simulink model "Task_Es"  (R2022b)
settings: Solver=ode45  StartTime=0.0  StopTime=10.0  RelTol=1e-3
undefined symbols (not defined in the file): A, absolute_encoder_counts_per_revolution, B, C, C_pid, Cz_zoh, init, Jgain, K_ctr_sine, K_I_sine, theta_l_init, vision_fps, w
libraries: simulink_extras x16
settings Model: Creator=tumisangramotlhwa  LastModifiedBy=tumisangramotlhwa

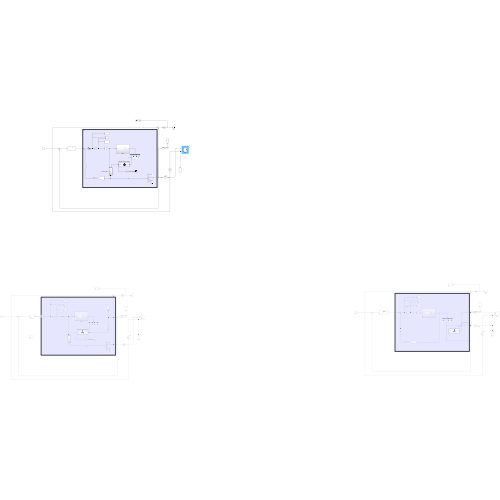
[thumbnail: Simulink's stored preview of the top-level diagram]
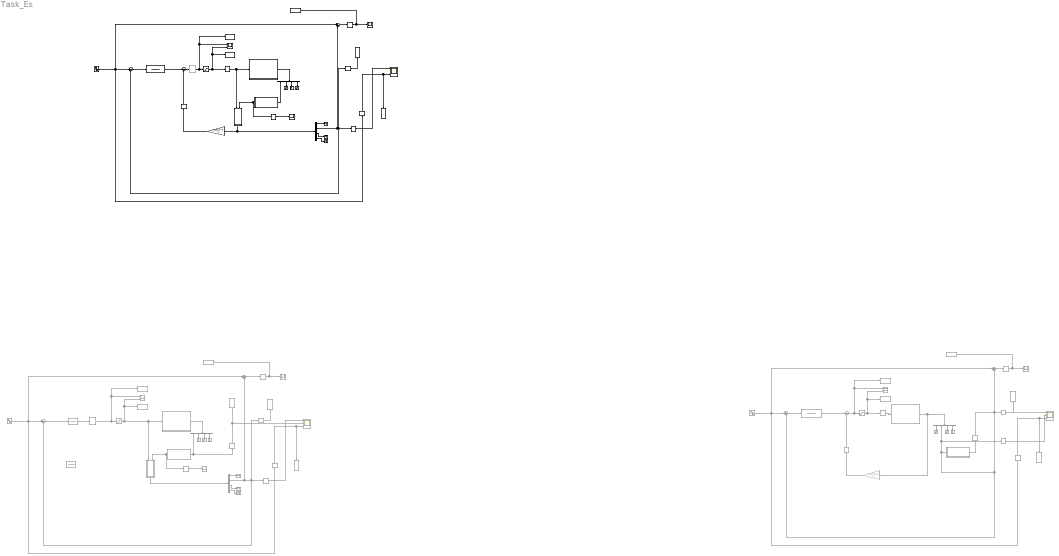
== system Task_Es ==
  note: G(s)
  note: G(s)
  note: G(s)
  AbsoluteEncoderSensorInterface1 : Subsystem  TreatAsAtomicUnit=on
      mask Display: image('$imagefile'); % Use "Edit Image" on toolstrip to change.
  AbsoluteEncoderSensorInterface2 : Subsystem  Commented=on  TreatAsAtomicUnit=on
      mask Display: image('$imagefile'); % Use "Edit Image" on toolstrip to change.
  C(s) : TransferFcn  Commented=on  Numerator=C_pid.Numerator{1,1}  Denominator=C_pid.Denominator{1,1}
  C(z) ZOH : DiscreteTransferFcn  Commented=on  Numerator=Cz_zoh.Numerator{1,1}  Denominator=Cz_zoh.Denominator{1,1}
  Demux1 : Demux
  Demux2 : Demux
  Demux3 : Demux  Commented=on
  Demux4 : Demux  Commented=on
  Demux5 : Demux  Commented=on
  K1 : Gain  Gain=K_ctr_sine  Multiplication=Matrix(K*u) (u vector)
  K2 : Gain  Commented=on  Gain=K_ctr_sine  Multiplication=Matrix(K*u) (u vector)
  Luenberger Observer : Subsystem  TreatAsAtomicUnit=on
  Luenberger Observer1 : Subsystem  Commented=on  TreatAsAtomicUnit=on
  Memory1 : Memory  Commented=on
  Memory2 : Memory
  Memory3 : Memory
  Memory4 : Memory  Commented=on
  PLANT1 : Subsystem
  PLANT2 : Subsystem  Commented=on
  PLANT3 : Subsystem  Commented=on
  Radians to Degrees{7..17} (11 alike) : simulink_extras/Transformations/Radians to Degrees  Commented=on
  Radians to Degrees{2..6} (5 alike) : simulink_extras/Transformations/Radians to Degrees
  Rate Transition : RateTransition  Commented=through  OutPortSampleTime=1/50
  Rate Transition1 : RateTransition  Commented=on  OutPortSampleTime=1/50
  Saturation1 : Saturate  UpperLimit=6  LowerLimit=-6
  Saturation2 : Saturate  Commented=on  UpperLimit=6  LowerLimit=-6
  Saturation3 : Saturate  Commented=on  UpperLimit=6  LowerLimit=-6
  Scope : Scope
  Scope1 : Scope  NumInputPorts=2
  Scope2 : Scope  Commented=on
  Scope3 : Scope  Commented=on  NumInputPorts=2
  Scope4 : Scope  Commented=on  NumInputPorts=2
  Sine Wave1 : Sin  Amplitude=deg2rad(20)  Frequency=pi/2  Phase=deg2rad(20)  SampleTime=0
  Sine Wave2 : Sin  Commented=on  Amplitude=deg2rad(20)  Frequency=pi/2  Phase=deg2rad(20)  SampleTime=0
  Sine Wave3 : Sin  Commented=on  Amplitude=deg2rad(20)  Frequency=pi/2  Phase=deg2rad(20)  SampleTime=0
  Sum{1,5,7..8} (4 alike) : Sum  Commented=on  Inputs=|+-
  Sum2 : Sum  Inputs=|+-
  Sum3 : Sum  Commented=on  Inputs=|--
  Sum4 : Sum  Inputs=|--
  Sum6 : Sum  Inputs=|+-
  Terminator{1..2,9..15} (9 alike) : Terminator  Commented=on
  Terminator{3..8} (6 alike) : Terminator
  To File1 : ToFile  Filename=Error.mat  MatrixName=Error  SaveFormat=Timeseries
  To File10 : ToFile  Commented=on  Filename=trueu.mat  MatrixName=trueu  SaveFormat=Timeseries
  To File11 : ToFile  Commented=on  Filename=truth.mat  MatrixName=truth  SaveFormat=Timeseries
  To File12 : ToFile  Commented=on  Filename=Error.mat  MatrixName=Error  SaveFormat=Timeseries
  To File13 : ToFile  Commented=on  Filename=reference.mat  MatrixName=reference  SaveFormat=Timeseries
  To File14 : ToFile  Commented=on  Filename=y.mat  MatrixName=y  SaveFormat=Timeseries
  To File15 : ToFile  Commented=on  Filename=commandu.mat  MatrixName=commandu  SaveFormat=Timeseries
  To File16 : ToFile  Commented=on  Filename=trueu.mat  MatrixName=trueu  SaveFormat=Timeseries
  To File2 : ToFile  Commented=on  Filename=Error.mat  MatrixName=Error  SaveFormat=Timeseries
  To File3 : ToFile  Commented=on  Filename=reference.mat  MatrixName=reference  SaveFormat=Timeseries
  To File4 : ToFile  Commented=on  Filename=y.mat  MatrixName=y  SaveFormat=Timeseries
  To File5 : ToFile  Commented=on  Filename=commandu.mat  MatrixName=commandu  SaveFormat=Timeseries
  To File6 : ToFile  Filename=reference.mat  MatrixName=reference  SaveFormat=Timeseries
  To File7 : ToFile  Filename=y.mat  MatrixName=y  SaveFormat=Timeseries
  To File8 : ToFile  Filename=commandu.mat  MatrixName=commandu  SaveFormat=Timeseries
  To File9 : ToFile  Filename=trueu.mat  MatrixName=trueu  SaveFormat=Timeseries
  Transfer Fcn : TransferFcn  Numerator=[K_I_sine]  Denominator=[1 0 w^2]
  Transfer Fcn1 : TransferFcn  Commented=on  Numerator=[K_I_sine]  Denominator=[1 0 w^2]
  VisionSensorInterface : Subsystem  Commented=on  TreatAsAtomicUnit=on
      mask Display: image('$imagefile'); % Use "Edit Image" on toolstrip to change.
  error1 : Scope  Commented=on
  error2 : Scope
  error3 : Scope  Commented=on
  scope1 : Scope  NumInputPorts=3
  scope2 : Scope  Commented=on  NumInputPorts=3
  scope3 : Scope  Commented=on  NumInputPorts=3
  wires:
  Luenberger Observer/1(x_hat) -> Demux2/1, K1/1  "x_hat"
  K1/1 -> Memory2/1  "K*x_hat"
  Memory3/1 -> Luenberger Observer/1(u), PLANT1/1(u)
  Demux2/4 -> Terminator7/1
  Transfer Fcn/1 -> Sum4/1
  PLANT1/1(x) -> Demux1/1
  Demux2/3 -> Terminator8/1
  Demux1/2 -> Terminator4/1
  Sum2/1 -> Transfer Fcn/1  "error"
  Memory2/1 -> Sum4/2
  Demux1/4 -> Terminator6/1
  Radians to Degrees5/1 -> scope1/3, To File6/1  "reference"
  Radians to Degrees4/1 -> To File7/1  "sensor measurement"
  Demux1/3 -> Terminator5/1
  Saturation1/1 -> Memory3/1, To File9/1, Scope1/2  "true input"
  Demux2/2 -> Radians to Degrees6/1, Radians to Degrees4/1, Sum2/2, Sum6/2  "link angle"
  Demux2/1 -> Terminator3/1
  Sum4/1 -> Rate Transition/1  "command input"
  Sine Wave1/1 -> Sum6/1, Radians to Degrees5/1, Sum2/1  "y"
  Radians to Degrees2/1 -> Scope/1  "sensor measurement"
  Radians to Degrees3/1 -> To File1/1, error2/1
  Sum6/1 -> Radians to Degrees3/1
  Radians to Degrees6/1 -> scope1/1  "link angle"
  K2/1 -> Memory1/1  "K*x_hat"
  PLANT2/1(x) -> Demux3/1, K2/1
  Demux3/3 -> Terminator9/1
  Demux3/4 -> Terminator10/1
  Sum5/1 -> Radians to Degrees9/1
  Radians to Degrees7/1 -> scope2/1  "sensor measurement"
  Radians to Degrees9/1 -> To File2/1, error1/1
  Transfer Fcn1/1 -> Sum3/1
  Saturation2/1 -> Memory4/1, To File10/1, Scope3/2  "true input"
  Sum3/1 -> Saturation2/1, To File5/1, Scope3/1  "command input"
  Sum1/1 -> Transfer Fcn1/1  "error"
  Radians to Degrees10/1 -> To File4/1  "sensor measurement"
  Memory1/1 -> Sum3/2
  Sine Wave2/1 -> Sum5/1, Radians to Degrees11/1, Sum1/1  "y"
  Demux3/2 -> Radians to Degrees8/1, Sum5/2, Radians to Degrees10/1, Sum1/2, VisionSensorInterface/1(y_plant)  "link angle"
  Memory4/1 -> PLANT2/1(u)
  Radians to Degrees11/1 -> scope2/3, To File3/1  "reference"
  Demux3/1 -> Terminator2/1
  VisionSensorInterface/1(y_vision) -> Radians to Degrees7/1
  Radians to Degrees8/1 -> scope2/2  "link angle"
  Rate Transition/1 -> Saturation1/1, To File8/1, Scope1/1
  AbsoluteEncoderSensorInterface1/1(y_absenc) -> Luenberger Observer/2(y), Radians to Degrees2/1
  Demux1/1 -> AbsoluteEncoderSensorInterface1/1(y_plant)
  Demux5/3 -> Terminator15/1
  Luenberger Observer1/1(x_hat) -> Demux5/1  "x_hat"
  AbsoluteEncoderSensorInterface2/1(y_absenc) -> Luenberger Observer1/2(y), Radians to Degrees13/1
  Radians to Degrees17/1 -> scope3/1  "link angle"
  Saturation3/1 -> Luenberger Observer1/1(u), PLANT3/1(u), To File16/1, Scope4/2  "true input"
  Radians to Degrees14/1 -> To File12/1, error3/1
  Demux5/2 -> Radians to Degrees17/1, Radians to Degrees15/1, Sum7/2, Sum8/2  "link angle"
  Radians to Degrees13/1 -> Scope2/1  "sensor measurement"
  Demux4/1 -> Radians to Degrees12/1, AbsoluteEncoderSensorInterface2/1(y_plant)
  PLANT3/1(x) -> Demux4/1
  Rate Transition1/1 -> Saturation3/1, To File15/1, Scope4/1
  Sum8/1 -> Radians to Degrees14/1
  Sine Wave3/1 -> Sum8/1, Radians to Degrees16/1, Sum7/1  "y"
  Demux5/4 -> Terminator14/1
  Demux4/2 -> Terminator11/1
  Demux4/4 -> Terminator13/1
  Demux4/3 -> Terminator12/1
  Radians to Degrees16/1 -> scope3/3, To File13/1  "reference"
  Radians to Degrees12/1 -> To File11/1, scope3/2  "ground truth"
  Demux5/1 -> Terminator1/1
  Radians to Degrees15/1 -> To File14/1  "sensor measurement"
  C(s)/1 -> Rate Transition1/1  "command input"
  Sum7/1 -> C(s)/1  "error"

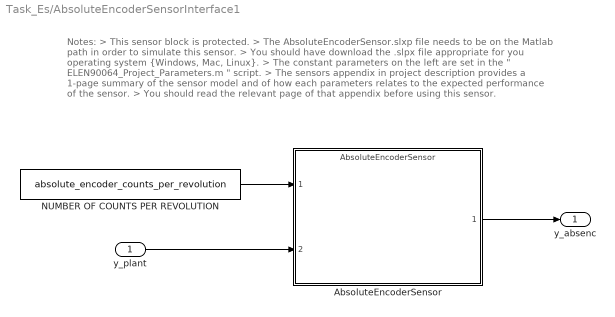
== system Task_Es/AbsoluteEncoderSensorInterface1 ==
  note: Notes:
      | > This sensor block is protected.
      | > The AbsoluteEncoderSensor.slxp file needs to be on the Matlab path in order to simulate this sensor.
      | > You should have download the .slpx file appropriate for you operating system {Windows, Mac, Linux}.
      | > The constant parameters on the left are set in the " ELEN90064_Project_Parameters.m " script.
      | > The sensors appendix in project description provides a 1-page summary of the sensor model and of how each parameters relates to the expected performance of the sensor.
      | > You should read the relevant page of that appendix before using this sensor.
  y_plant : Inport
  AbsoluteEncoderSensor : ModelReference  ModelNameDialog=AbsoluteEncoderSensor.slxp  ModelReferenceVersion=1.16  CopyOfModelProtected=on
  NUMBER OF COUNTS PER REVOLUTION : Constant  Value=absolute_encoder_counts_per_revolution
  y_absenc : Outport
  wires:
  NUMBER OF COUNTS PER REVOLUTION/1 -> AbsoluteEncoderSensor/1
  y_plant/1 -> AbsoluteEncoderSensor/2
  AbsoluteEncoderSensor/1 -> y_absenc/1

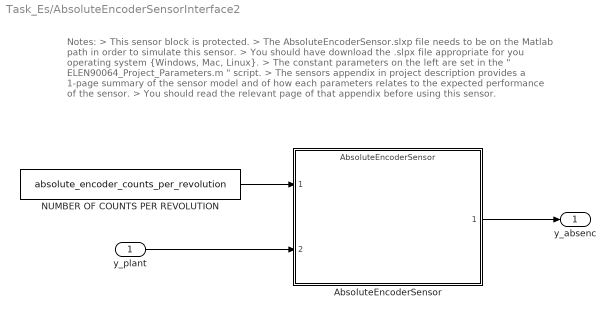
== system Task_Es/AbsoluteEncoderSensorInterface2 ==
  note: Notes:
      | > This sensor block is protected.
      | > The AbsoluteEncoderSensor.slxp file needs to be on the Matlab path in order to simulate this sensor.
      | > You should have download the .slpx file appropriate for you operating system {Windows, Mac, Linux}.
      | > The constant parameters on the left are set in the " ELEN90064_Project_Parameters.m " script.
      | > The sensors appendix in project description provides a 1-page summary of the sensor model and of how each parameters relates to the expected performance of the sensor.
      | > You should read the relevant page of that appendix before using this sensor.
  y_plant : Inport
  AbsoluteEncoderSensor : ModelReference  ModelNameDialog=AbsoluteEncoderSensor.slxp  ModelReferenceVersion=1.16  CopyOfModelProtected=on
  NUMBER OF COUNTS PER REVOLUTION : Constant  Value=absolute_encoder_counts_per_revolution
  y_absenc : Outport
  wires:
  NUMBER OF COUNTS PER REVOLUTION/1 -> AbsoluteEncoderSensor/1
  y_plant/1 -> AbsoluteEncoderSensor/2
  AbsoluteEncoderSensor/1 -> y_absenc/1

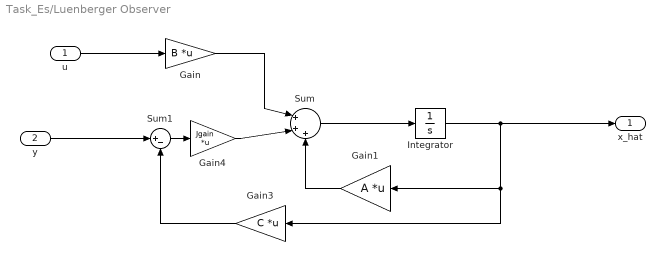
== system Task_Es/Luenberger Observer ==
  u : Inport
  y : Inport  Port=2
  Gain : Gain  Gain=B  Multiplication=Matrix(K*u) (u vector)
  Gain1 : Gain  Gain=A  Multiplication=Matrix(K*u) (u vector)
  Gain3 : Gain  Gain=C  Multiplication=Matrix(K*u) (u vector)
  Gain4 : Gain  Gain=Jgain  Multiplication=Matrix(K*u) (u vector)
  Integrator : Integrator
  Sum : Sum  Inputs=|+++
  Sum1 : Sum  Inputs=|+-
  x_hat : Outport
  wires:
  Gain/1 -> Sum/1
  Gain4/1 -> Sum/2
  Sum1/1 -> Gain4/1
  Gain3/1 -> Sum1/2
  Gain1/1 -> Sum/3
  Sum/1 -> Integrator/1
  Integrator/1 -> x_hat/1, Gain1/1, Gain3/1
  u/1 -> Gain/1
  y/1 -> Sum1/1

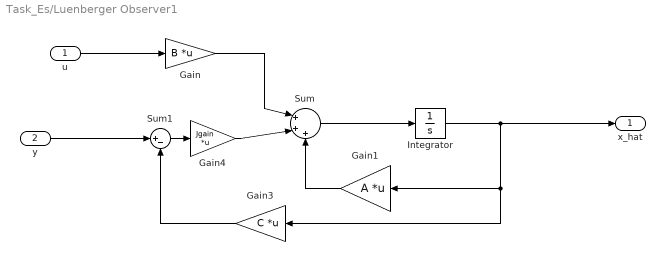
== system Task_Es/Luenberger Observer1 ==
  u : Inport
  y : Inport  Port=2
  Gain : Gain  Gain=B  Multiplication=Matrix(K*u) (u vector)
  Gain1 : Gain  Gain=A  Multiplication=Matrix(K*u) (u vector)
  Gain3 : Gain  Gain=C  Multiplication=Matrix(K*u) (u vector)
  Gain4 : Gain  Gain=Jgain  Multiplication=Matrix(K*u) (u vector)
  Integrator : Integrator
  Sum : Sum  Inputs=|+++
  Sum1 : Sum  Inputs=|+-
  x_hat : Outport
  wires:
  Gain/1 -> Sum/1
  Gain4/1 -> Sum/2
  Sum1/1 -> Gain4/1
  Gain3/1 -> Sum1/2
  Gain1/1 -> Sum/3
  Sum/1 -> Integrator/1
  Integrator/1 -> x_hat/1, Gain1/1, Gain3/1
  u/1 -> Gain/1
  y/1 -> Sum1/1

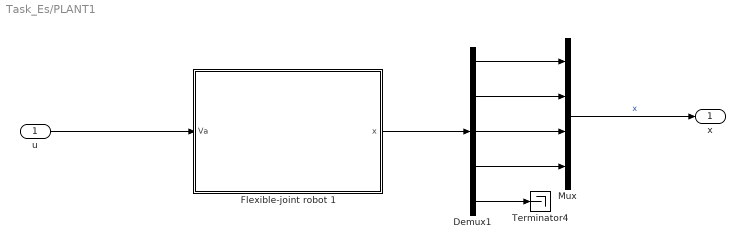
== system Task_Es/PLANT1 ==
  u : Inport
  Demux1 : Demux  Outputs=5
  Flexible-joint robot 1 : Subsystem
      mask Display: image('$imagefile'); % Use "Edit Image" on toolstrip to change.
  Mux : Mux
  Terminator4 : Terminator
  x : Outport
  wires:
  Mux/1 -> x/1  "x"
  Demux1/4 -> Mux/4
  Flexible-joint robot 1/1(x) -> Demux1/1
  Demux1/3 -> Mux/3
  Demux1/2 -> Mux/2
  Demux1/1 -> Mux/1
  Demux1/5 -> Terminator4/1
  u/1 -> Flexible-joint robot 1/1(Va)

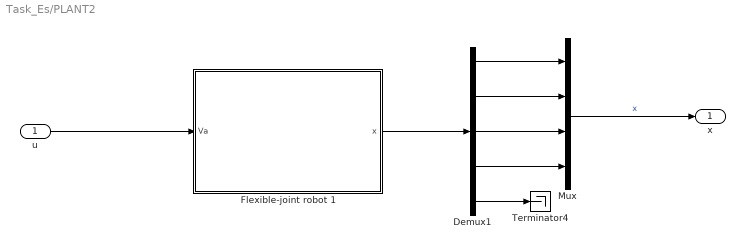
== system Task_Es/PLANT2 ==
  u : Inport
  Demux1 : Demux  Outputs=5
  Flexible-joint robot 1 : Subsystem
      mask Display: image('$imagefile'); % Use "Edit Image" on toolstrip to change.
  Mux : Mux
  Terminator4 : Terminator
  x : Outport
  wires:
  Mux/1 -> x/1  "x"
  Demux1/4 -> Mux/4
  Flexible-joint robot 1/1(x) -> Demux1/1
  Demux1/3 -> Mux/3
  Demux1/2 -> Mux/2
  Demux1/1 -> Mux/1
  Demux1/5 -> Terminator4/1
  u/1 -> Flexible-joint robot 1/1(Va)

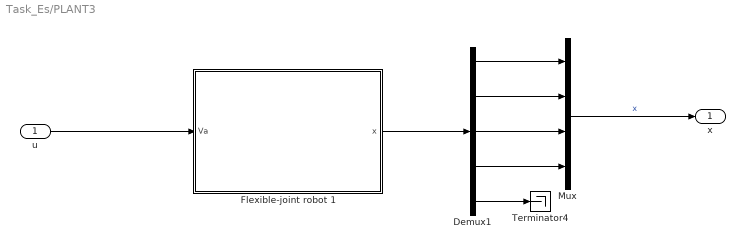
== system Task_Es/PLANT3 ==
  u : Inport
  Demux1 : Demux  Outputs=5
  Flexible-joint robot 1 : Subsystem
      mask Display: image('$imagefile'); % Use "Edit Image" on toolstrip to change.
  Mux : Mux
  Terminator4 : Terminator
  x : Outport
  wires:
  Mux/1 -> x/1  "x"
  Demux1/4 -> Mux/4
  Flexible-joint robot 1/1(x) -> Demux1/1
  Demux1/3 -> Mux/3
  Demux1/2 -> Mux/2
  Demux1/1 -> Mux/1
  Demux1/5 -> Terminator4/1
  u/1 -> Flexible-joint robot 1/1(Va)

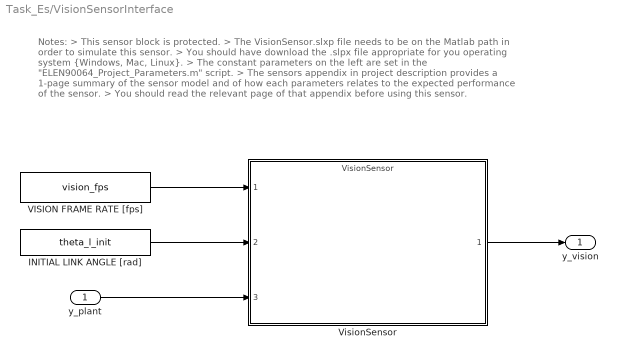
== system Task_Es/VisionSensorInterface ==
  note: Notes:
      | > This sensor block is protected.
      | > The VisionSensor.slxp file needs to be on the Matlab path in order to simulate this sensor.
      | > You should have download the .slpx file appropriate for you operating system {Windows, Mac, Linux}.
      | > The constant parameters on the left are set in the "ELEN90064_Project_Parameters.m" script.
      | > The sensors appendix in project description provides a 1-page summary of the sensor model and of how each parameters relates to the expected performance of the sensor.
      | > You should read the relevant page of that appendix before using this sensor.
  y_plant : Inport
  INITIAL LINK ANGLE [rad] : Constant  Value=theta_l_init
  VISION FRAME RATE [fps] : Constant  Value=vision_fps
  VisionSensor : ModelReference  ModelNameDialog=VisionSensor.slxp  ModelReferenceVersion=1.19  CopyOfModelProtected=on
  y_vision : Outport
  wires:
  VISION FRAME RATE [fps]/1 -> VisionSensor/1
  INITIAL LINK ANGLE [rad]/1 -> VisionSensor/2
  y_plant/1 -> VisionSensor/3
  VisionSensor/1 -> y_vision/1

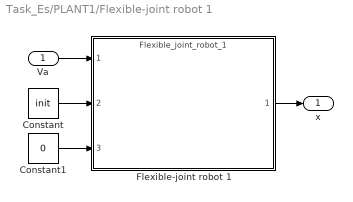
== system Task_Es/PLANT1/Flexible-joint robot 1 ==
  Va : Inport
  Constant : Constant  Value=init
  Constant1 : Constant  Value=0
  Flexible-joint robot 1 : ModelReference  ModelNameDialog=Flexible_joint_robot_1  ModelReferenceVersion=1.63  CopyOfModelProtected=on
  x : Outport
  wires:
  Constant/1 -> Flexible-joint robot 1/2
  Constant1/1 -> Flexible-joint robot 1/3
  Flexible-joint robot 1/1 -> x/1
  Va/1 -> Flexible-joint robot 1/1

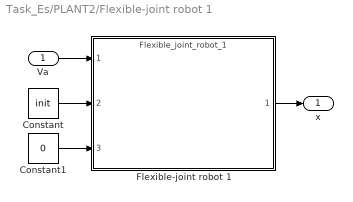
== system Task_Es/PLANT2/Flexible-joint robot 1 ==
  Va : Inport
  Constant : Constant  Value=init
  Constant1 : Constant  Value=0
  Flexible-joint robot 1 : ModelReference  ModelNameDialog=Flexible_joint_robot_1  ModelReferenceVersion=1.63  CopyOfModelProtected=on
  x : Outport
  wires:
  Constant/1 -> Flexible-joint robot 1/2
  Constant1/1 -> Flexible-joint robot 1/3
  Flexible-joint robot 1/1 -> x/1
  Va/1 -> Flexible-joint robot 1/1

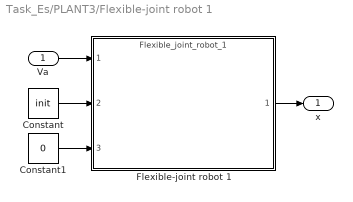
== system Task_Es/PLANT3/Flexible-joint robot 1 ==
  Va : Inport
  Constant : Constant  Value=init
  Constant1 : Constant  Value=0
  Flexible-joint robot 1 : ModelReference  ModelNameDialog=Flexible_joint_robot_1  ModelReferenceVersion=1.63  CopyOfModelProtected=on
  x : Outport
  wires:
  Constant/1 -> Flexible-joint robot 1/2
  Constant1/1 -> Flexible-joint robot 1/3
  Flexible-joint robot 1/1 -> x/1
  Va/1 -> Flexible-joint robot 1/1
